simulink library "csc_tdl_thruster_dynamics_collection_mtv_lib"  (R2014b)
settings: Solver=ode45  StartTime=0.0  StopTime=10.0  RelTol=1e-3
libraries: csu_tdl_thruster_dynamics_lander_lib x12, util_info_lib x1
settings Model: Creator=escrane  LastModifiedBy=mstewart

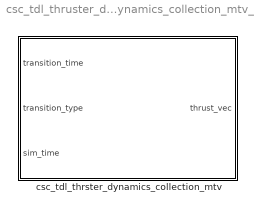
== system csc_tdl_thruster_dynamics_collection_mtv_lib ==
  csc_tdl_thrster_dynamics_collection_mtv : Subsystem
      mask Display: color('blue');text(0.05, 0.02, 'MoonEx', 'HorizontalAlignment', 'Left', 'VerticalAlignment', 'Bottom');color('red');text(0.95, 0.02, 'Autogenerated', 'HorizontalAlignment', 'Right', 'VerticalAlignment', 'Bottom');

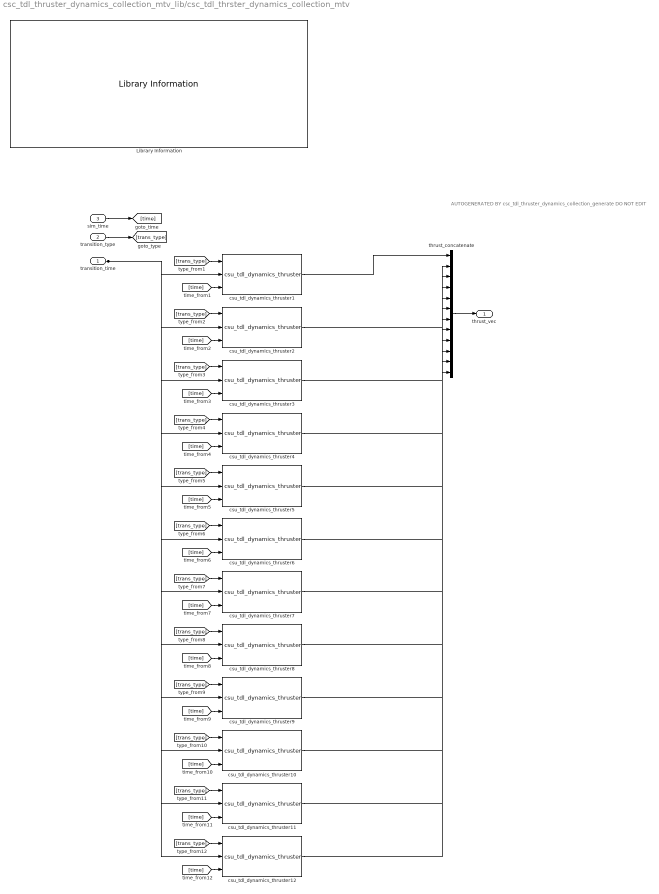
== system csc_tdl_thruster_dynamics_collection_mtv_lib/csc_tdl_thrster_dynamics_collection_mtv ==
  note: AUTOGENERATED BY csc_tdl_thruster_dynamics_collection_generate
      | DO NOT EDIT
  transition_time : Inport
  transition_type : Inport  Port=2
  sim_time : Inport  Port=3
  Library Information : util_info_lib/Library Information  owner='NONE'
  csu_tdl_dynamics_thruster1 : csu_tdl_thruster_dynamics_lander_lib/csu_tdl_dynamics_thruster  thruster_idx=1  num_thrusters=12  time_since_rise_lookup=tdl_thruster1_rising_lookup_time  thrust_rising_output_lookup=tdl_thruster1_rising_lookup_thrust  time_since_fall_lookup=tdl_thruster1_falling_lookup_time  thrust_falling_output_lookup=tdl_thruster1_falling_lookup_thrust  thrust_noise_mean=tdl_thruster1_thrust_noise_mean  thrust_noise_std=tdl_thruster1_thrust_noise_std  thrust_noise_seed=tdl_thruster1_thrust_noise_seed  thrust_noise_on=tdl_thruster1_thrust_noise_enable
  csu_tdl_dynamics_thruster10 : csu_tdl_thruster_dynamics_lander_lib/csu_tdl_dynamics_thruster  thruster_idx=10  num_thrusters=12  time_since_rise_lookup=tdl_thruster10_rising_lookup_time  thrust_rising_output_lookup=tdl_thruster10_rising_lookup_thrust  time_since_fall_lookup=tdl_thruster10_falling_lookup_time  thrust_falling_output_lookup=tdl_thruster10_falling_lookup_thrust  thrust_noise_mean=tdl_thruster10_thrust_noise_mean  thrust_noise_std=tdl_thruster10_thrust_noise_std  thrust_noise_seed=tdl_thruster10_thrust_noise_seed  thrust_noise_on=tdl_thruster10_thrust_noise_enable
  csu_tdl_dynamics_thruster11 : csu_tdl_thruster_dynamics_lander_lib/csu_tdl_dynamics_thruster  thruster_idx=11  num_thrusters=12  time_since_rise_lookup=tdl_thruster11_rising_lookup_time  thrust_rising_output_lookup=tdl_thruster11_rising_lookup_thrust  time_since_fall_lookup=tdl_thruster11_falling_lookup_time  thrust_falling_output_lookup=tdl_thruster11_falling_lookup_thrust  thrust_noise_mean=tdl_thruster11_thrust_noise_mean  thrust_noise_std=tdl_thruster11_thrust_noise_std  thrust_noise_seed=tdl_thruster11_thrust_noise_seed  thrust_noise_on=tdl_thruster11_thrust_noise_enable
  csu_tdl_dynamics_thruster12 : csu_tdl_thruster_dynamics_lander_lib/csu_tdl_dynamics_thruster  thruster_idx=12  num_thrusters=12  time_since_rise_lookup=tdl_thruster12_rising_lookup_time  thrust_rising_output_lookup=tdl_thruster12_rising_lookup_thrust  time_since_fall_lookup=tdl_thruster12_falling_lookup_time  thrust_falling_output_lookup=tdl_thruster12_falling_lookup_thrust  thrust_noise_mean=tdl_thruster12_thrust_noise_mean  thrust_noise_std=tdl_thruster12_thrust_noise_std  thrust_noise_seed=tdl_thruster12_thrust_noise_seed  thrust_noise_on=tdl_thruster12_thrust_noise_enable
  csu_tdl_dynamics_thruster2 : csu_tdl_thruster_dynamics_lander_lib/csu_tdl_dynamics_thruster  thruster_idx=2  num_thrusters=12  time_since_rise_lookup=tdl_thruster2_rising_lookup_time  thrust_rising_output_lookup=tdl_thruster2_rising_lookup_thrust  time_since_fall_lookup=tdl_thruster2_falling_lookup_time  thrust_falling_output_lookup=tdl_thruster2_falling_lookup_thrust  thrust_noise_mean=tdl_thruster2_thrust_noise_mean  thrust_noise_std=tdl_thruster2_thrust_noise_std  thrust_noise_seed=tdl_thruster2_thrust_noise_seed  thrust_noise_on=tdl_thruster2_thrust_noise_enable
  csu_tdl_dynamics_thruster3 : csu_tdl_thruster_dynamics_lander_lib/csu_tdl_dynamics_thruster  thruster_idx=3  num_thrusters=12  time_since_rise_lookup=tdl_thruster3_rising_lookup_time  thrust_rising_output_lookup=tdl_thruster3_rising_lookup_thrust  time_since_fall_lookup=tdl_thruster3_falling_lookup_time  thrust_falling_output_lookup=tdl_thruster3_falling_lookup_thrust  thrust_noise_mean=tdl_thruster3_thrust_noise_mean  thrust_noise_std=tdl_thruster3_thrust_noise_std  thrust_noise_seed=tdl_thruster3_thrust_noise_seed  thrust_noise_on=tdl_thruster3_thrust_noise_enable
  csu_tdl_dynamics_thruster4 : csu_tdl_thruster_dynamics_lander_lib/csu_tdl_dynamics_thruster  thruster_idx=4  num_thrusters=12  time_since_rise_lookup=tdl_thruster4_rising_lookup_time  thrust_rising_output_lookup=tdl_thruster4_rising_lookup_thrust  time_since_fall_lookup=tdl_thruster4_falling_lookup_time  thrust_falling_output_lookup=tdl_thruster4_falling_lookup_thrust  thrust_noise_mean=tdl_thruster4_thrust_noise_mean  thrust_noise_std=tdl_thruster4_thrust_noise_std  thrust_noise_seed=tdl_thruster4_thrust_noise_seed  thrust_noise_on=tdl_thruster4_thrust_noise_enable
  csu_tdl_dynamics_thruster5 : csu_tdl_thruster_dynamics_lander_lib/csu_tdl_dynamics_thruster  thruster_idx=5  num_thrusters=12  time_since_rise_lookup=tdl_thruster5_rising_lookup_time  thrust_rising_output_lookup=tdl_thruster5_rising_lookup_thrust  time_since_fall_lookup=tdl_thruster5_falling_lookup_time  thrust_falling_output_lookup=tdl_thruster5_falling_lookup_thrust  thrust_noise_mean=tdl_thruster5_thrust_noise_mean  thrust_noise_std=tdl_thruster5_thrust_noise_std  thrust_noise_seed=tdl_thruster5_thrust_noise_seed  thrust_noise_on=tdl_thruster5_thrust_noise_enable
  csu_tdl_dynamics_thruster6 : csu_tdl_thruster_dynamics_lander_lib/csu_tdl_dynamics_thruster  thruster_idx=6  num_thrusters=12  time_since_rise_lookup=tdl_thruster6_rising_lookup_time  thrust_rising_output_lookup=tdl_thruster6_rising_lookup_thrust  time_since_fall_lookup=tdl_thruster6_falling_lookup_time  thrust_falling_output_lookup=tdl_thruster6_falling_lookup_thrust  thrust_noise_mean=tdl_thruster6_thrust_noise_mean  thrust_noise_std=tdl_thruster6_thrust_noise_std  thrust_noise_seed=tdl_thruster6_thrust_noise_seed  thrust_noise_on=tdl_thruster6_thrust_noise_enable
  csu_tdl_dynamics_thruster7 : csu_tdl_thruster_dynamics_lander_lib/csu_tdl_dynamics_thruster  thruster_idx=7  num_thrusters=12  time_since_rise_lookup=tdl_thruster7_rising_lookup_time  thrust_rising_output_lookup=tdl_thruster7_rising_lookup_thrust  time_since_fall_lookup=tdl_thruster7_falling_lookup_time  thrust_falling_output_lookup=tdl_thruster7_falling_lookup_thrust  thrust_noise_mean=tdl_thruster7_thrust_noise_mean  thrust_noise_std=tdl_thruster7_thrust_noise_std  thrust_noise_seed=tdl_thruster7_thrust_noise_seed  thrust_noise_on=tdl_thruster7_thrust_noise_enable
  csu_tdl_dynamics_thruster8 : csu_tdl_thruster_dynamics_lander_lib/csu_tdl_dynamics_thruster  thruster_idx=8  num_thrusters=12  time_since_rise_lookup=tdl_thruster8_rising_lookup_time  thrust_rising_output_lookup=tdl_thruster8_rising_lookup_thrust  time_since_fall_lookup=tdl_thruster8_falling_lookup_time  thrust_falling_output_lookup=tdl_thruster8_falling_lookup_thrust  thrust_noise_mean=tdl_thruster8_thrust_noise_mean  thrust_noise_std=tdl_thruster8_thrust_noise_std  thrust_noise_seed=tdl_thruster8_thrust_noise_seed  thrust_noise_on=tdl_thruster8_thrust_noise_enable
  csu_tdl_dynamics_thruster9 : csu_tdl_thruster_dynamics_lander_lib/csu_tdl_dynamics_thruster  thruster_idx=9  num_thrusters=12  time_since_rise_lookup=tdl_thruster9_rising_lookup_time  thrust_rising_output_lookup=tdl_thruster9_rising_lookup_thrust  time_since_fall_lookup=tdl_thruster9_falling_lookup_time  thrust_falling_output_lookup=tdl_thruster9_falling_lookup_thrust  thrust_noise_mean=tdl_thruster9_thrust_noise_mean  thrust_noise_std=tdl_thruster9_thrust_noise_std  thrust_noise_seed=tdl_thruster9_thrust_noise_seed  thrust_noise_on=tdl_thruster9_thrust_noise_enable
  thrust_concatenate : Concatenate  NumInputs=12
  thrust_vec : Outport
  wires:
  sim_time/1 -> [time]
  transition_type/1 -> [trans_type]
  thrust_concatenate/1 -> thrust_vec/1
  [time] -> csu_tdl_dynamics_thruster1/3
  [trans_type] -> csu_tdl_dynamics_thruster1/1
  csu_tdl_dynamics_thruster1/1 -> thrust_concatenate/1
  [time] -> csu_tdl_dynamics_thruster2/3
  [trans_type] -> csu_tdl_dynamics_thruster2/1
  csu_tdl_dynamics_thruster2/1 -> thrust_concatenate/2
  [time] -> csu_tdl_dynamics_thruster3/3
  [trans_type] -> csu_tdl_dynamics_thruster3/1
  csu_tdl_dynamics_thruster3/1 -> thrust_concatenate/3
  [time] -> csu_tdl_dynamics_thruster4/3
  [trans_type] -> csu_tdl_dynamics_thruster4/1
  csu_tdl_dynamics_thruster4/1 -> thrust_concatenate/4
  [time] -> csu_tdl_dynamics_thruster5/3
  [trans_type] -> csu_tdl_dynamics_thruster5/1
  csu_tdl_dynamics_thruster5/1 -> thrust_concatenate/5
  [time] -> csu_tdl_dynamics_thruster6/3
  [trans_type] -> csu_tdl_dynamics_thruster6/1
  csu_tdl_dynamics_thruster6/1 -> thrust_concatenate/6
  [time] -> csu_tdl_dynamics_thruster7/3
  [trans_type] -> csu_tdl_dynamics_thruster7/1
  csu_tdl_dynamics_thruster7/1 -> thrust_concatenate/7
  [time] -> csu_tdl_dynamics_thruster8/3
  [trans_type] -> csu_tdl_dynamics_thruster8/1
  csu_tdl_dynamics_thruster8/1 -> thrust_concatenate/8
  [time] -> csu_tdl_dynamics_thruster9/3
  [trans_type] -> csu_tdl_dynamics_thruster9/1
  csu_tdl_dynamics_thruster9/1 -> thrust_concatenate/9
  [time] -> csu_tdl_dynamics_thruster10/3
  [trans_type] -> csu_tdl_dynamics_thruster10/1
  csu_tdl_dynamics_thruster10/1 -> thrust_concatenate/10
  [time] -> csu_tdl_dynamics_thruster11/3
  [trans_type] -> csu_tdl_dynamics_thruster11/1
  csu_tdl_dynamics_thruster11/1 -> thrust_concatenate/11
  [time] -> csu_tdl_dynamics_thruster12/3
  [trans_type] -> csu_tdl_dynamics_thruster12/1
  csu_tdl_dynamics_thruster12/1 -> thrust_concatenate/12
  transition_time/1 -> csu_tdl_dynamics_thruster12/2, csu_tdl_dynamics_thruster11/2, csu_tdl_dynamics_thruster10/2, csu_tdl_dynamics_thruster9/2, csu_tdl_dynamics_thruster8/2, csu_tdl_dynamics_thruster7/2, csu_tdl_dynamics_thruster6/2, csu_tdl_dynamics_thruster5/2, csu_tdl_dynamics_thruster4/2, csu_tdl_dynamics_thruster3/2, csu_tdl_dynamics_thruster2/2, csu_tdl_dynamics_thruster1/2
